simulink model "verify_StorageType3_mdl"  (R2016b)
settings: Solver=ode45  StartTime=0.0  StopTime=24*3600  MaxStep=900  RelTol=1e-3  EnableMultiTasking=on
libraries: carnot x7
settings Model: Creator=drhf  LastModifiedBy=drhf
settings DataIOCC: SaveFormat=Array
settings OptimizationCC: ExpressionDepthLimit=2147483647  LifeSpan=inf
settings DebuggingCC: UnderspecifiedInitializationDetection=Classic  MergeDetectMultiDrivingBlocksExec=none  SolverPrmCheckMsg=warning  StateNameClashWarn=warning  SFUnexpectedBacktrackingDiag=warning  SFNoUnconditionalDefaultTransitionDiag=warning  SFExecutionAtInitializationDiag=none
settings HardwareCC: ProdBitPerPointer=32  ProdBitPerSizeT=32  ProdBitPerPtrDiffT=32  ProdLargestAtomicFloat=None  ProdIntDivRoundTo=Undefined  ProdEndianess=Unspecified  ProdWordSize=32  ProdHWDeviceType=32-bit Generic
settings ModelReferenceCC: PropagateSignalLabelsOutOfModel=off
settings GRTTargetCC: TargetLangStandard=C89/C90 (ANSI)  GeneratePreprocessorConditionals=Disable all  CombineOutputUpdateFcns=off  GRTInterface=on
settings ConfigComp: CovMetricSettings=dw  CovHtmlReporting=on  CovSaveCumulativeToWorkspaceVar=on  CovSaveSingleToWorkspaceVar=on  CovExternalEMLEnable=off

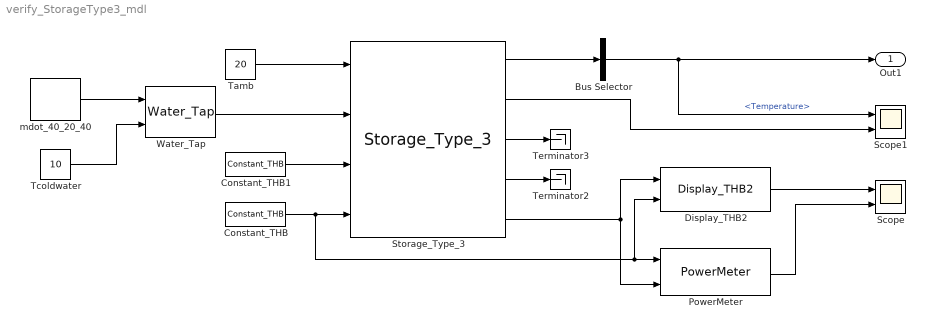
== system verify_StorageType3_mdl ==
  Bus Selector : BusSelector  OutputSignals=THBout_pipe1.Temperature
  Constant_THB : carnot/Source/Simple/Constant_THB  t=50  mdot=200/3600  p=1e5  mID=No Pressure Drop  fluid=Water (Constant 20°C)  mix=0  mix2=0  mix3=0  dia=0.02  hgt=0
  Constant_THB1 : carnot/Source/Simple/Constant_THB  t=60  mdot=600/3600  p=1e5  mID=No Pressure Drop  fluid=Water (Constant 20°C)  mix=0  mix2=0  mix3=0  dia=0.02  hgt=0
  Display_THB2 : carnot/Outputs/Display_THB2  t=on  m=off  p=off  id=off  mix=off  d=off
  PowerMeter : carnot/Control/PowerMeter
  Scope : Scope  NumInputPorts=2
  Scope1 : Scope  NumInputPorts=2
  Storage_Type_3 : carnot/Storage/Thermal/Storage_Type_3  uloss=1  ubot=1  utop=1  cond=1  volume=0.3  dia=0.5  pos=standing cylinder  h_in_hxup=0.81  h_out_hxup=0.56  ua0_hxup=80  uam_hxup=0.2  uat_hxup=0.5  dplin_hxup=100  dpqua_hxup=100  h_in_hxlw=0.48  h_out_hxlw=0.04  ua0_hxlw=100  uam_hxlw=0.2  uat_hxlw=0.5  dplin_hxlw=100  dpqua_hxlw=100  h_in=0  h_out=1  diapipe=0.04  t0=[10:5:55]  nodes=10  mpoints=10
  Tamb : Constant  Value=20
  Tcoldwater : Constant  Value=10
  Terminator2 : Terminator
  Terminator3 : Terminator
  Water_Tap : carnot/Load/Hot_Water_Tapping/Water_Tap  dia=0.02  p=2e5
  mdot_40_20_40 : carnot/Load/Hot_Water_Tapping/mdot_40_20_40  period=24*3600  rep_seq_t=[7 12 19]*3600  rep_seq_d=[0.2 0.1 0.2]*3600  rep_seq_y=[1 1 1]*200/1800
  Out1 : Outport
  wires:
  Tamb/1 -> Storage_Type_3/1
  Storage_Type_3/3 -> Terminator3/1
  Storage_Type_3/4 -> Terminator2/1
  Storage_Type_3/5 -> PowerMeter/2, Display_THB2/1
  Constant_THB1/1 -> Storage_Type_3/3
  Display_THB2/1 -> Scope/1
  Constant_THB/1 -> Storage_Type_3/4, PowerMeter/1, Display_THB2/2
  PowerMeter/1 -> Scope/2
  Water_Tap/1 -> Storage_Type_3/2
  mdot_40_20_40/1 -> Water_Tap/1
  Tcoldwater/1 -> Water_Tap/2
  Storage_Type_3/2 -> Scope1/2
  Storage_Type_3/1 -> Bus Selector/1
  Bus Selector/1 -> Scope1/1, Out1/1  "<Temperature>"
